simulink model "Experiment1_model"  (R2022a)
settings: Solver=FixedStepAuto  StartTime=0.0  StopTime=20  RelTol=1e-3
libraries: slpidlib x32, slctrlblks x18
(part 5 of 5)

== matlab function Experiment1_model/Safety CBF Enforcement Decentralized with Neighbours /CBF Robot5/Neighbourhood Radius ==
  data: hx5 input; hx5 output; qx5 input; deltaP5 input; qx5 output
function [hx5, qx5] = fcn(hx5, qx5, deltaP5)

E = 7;         % Maximum number of barriers
Ds = 0.6;      % Safe Distance
gamma = 0.3;   % Neighbour radius parameter 

Dn5 = Ds + 1/(2*(10+10)) * ((2*(10+10)/gamma)^(1/2) + (2+2))^2;

for i=1:E
    if deltaP5(i) >= Dn5
        hx5(i) = 0;
        qx5(i,:) = 0;
    end
end

== matlab function Experiment1_model/Safety CBF Enforcement Decentralized with Neighbours /CBF Robot6/DeltaP ==
  data: states input; deltaP6 output
function deltaP6 = fcn(states)

p1 = states(1:2);
p2 = states(3:4);
p3 = states(5:6);
p4 = states(7:8);
p5 = states(9:10);
p6 = states(11:12);
p7 = states(13:14);
p8 = states(15:16);

v1 = states(17:18);
v2 = states(19:20);
v3 = states(21:22);
v4 = states(23:24);
v5 = states(25:26);
v6 = states(27:28);
v7 = states(29:30);
v8 = states(31:32);

deltaP6 = CBF8Robots_deltaP6(states);

== matlab function Experiment1_model/Safety CBF Enforcement Decentralized with Neighbours /CBF Robot6/Neighbourhood Radius ==
  data: hx6 input; hx6 output; qx6 input; deltaP6 input; qx6 output
function [hx6, qx6] = fcn(hx6, qx6, deltaP6)

E = 7;         % Maximum number of barriers
Ds = 0.6;      % Safe Distance
gamma = 0.3;   % Neighbour radius parameter 

Dn6 = Ds + 1/(2*(10+10)) * ((2*(10+10)/gamma)^(1/2) + (2+2))^2;

for i=1:E
    if deltaP6(i) >= Dn6
        hx6(i) = 0;
        qx6(i,:) = 0;
    end
end

== matlab function Experiment1_model/Safety CBF Enforcement Decentralized with Neighbours /CBF Robot7/DeltaP ==
  data: states input; deltaP7 output
function deltaP7 = fcn(states)

p1 = states(1:2);
p2 = states(3:4);
p3 = states(5:6);
p4 = states(7:8);
p5 = states(9:10);
p6 = states(11:12);
p7 = states(13:14);
p8 = states(15:16);

v1 = states(17:18);
v2 = states(19:20);
v3 = states(21:22);
v4 = states(23:24);
v5 = states(25:26);
v6 = states(27:28);
v7 = states(29:30);
v8 = states(31:32);

deltaP7 = CBF8Robots_deltaP7(states);

== matlab function Experiment1_model/Safety CBF Enforcement Decentralized with Neighbours /CBF Robot7/Neighbourhood Radius ==
  data: hx7 input; hx7 output; qx7 input; deltaP7 input; qx7 output
function [hx7, qx7] = fcn(hx7, qx7, deltaP7)

E = 7;         % Maximum number of barriers
Ds = 0.6;      % Safe Distance
gamma = 0.3;   % Neighbour radius parameter 

Dn7 = Ds + 1/(2*(10+10)) * ((2*(10+10)/gamma)^(1/2) + (2+2))^2;

for i=1:E
    if deltaP7(i) >= Dn7
        hx7(i) = 0;
        qx7(i,:) = 0;
    end
end

== matlab function Experiment1_model/Safety CBF Enforcement Decentralized with Neighbours /CBF Robot8/DeltaP ==
  data: states input; deltaP8 output
function deltaP8 = fcn(states)

p1 = states(1:2);
p2 = states(3:4);
p3 = states(5:6);
p4 = states(7:8);
p5 = states(9:10);
p6 = states(11:12);
p7 = states(13:14);
p8 = states(15:16);

v1 = states(17:18);
v2 = states(19:20);
v3 = states(21:22);
v4 = states(23:24);
v5 = states(25:26);
v6 = states(27:28);
v7 = states(29:30);
v8 = states(31:32);

deltaP8 = CBF8Robots_deltaP8(states);

== matlab function Experiment1_model/Safety CBF Enforcement Decentralized with Neighbours /CBF Robot8/Neighbourhood Radius ==
  data: hx8 input; hx8 output; qx8 input; deltaP8 input; qx8 output
function [hx8, qx8] = fcn(hx8, qx8, deltaP8)

E = 7;         % Maximum number of barriers
Ds = 0.6;      % Safe Distance
gamma = 0.3;   % Neighbour radius parameter 

Dn8 = Ds + 1/(2*(10+10)) * ((2*(10+10)/gamma)^(1/2) + (2+2))^2;

for i=1:E
    if deltaP8(i) >= Dn8
        hx8(i) = 0;
        qx8(i,:) = 0;
    end
end

== matlab function Experiment1_model/Safety CBF Enforcement Decentralized with Neighbours /CBF Robot8/dh ==
  data: states input size=32; qx8 output size=[7 4]
function qx8 = fcn(states)
p1 = states(1:2);
p2 = states(3:4);
p3 = states(5:6);
p4 = states(7:8);
p5 = states(9:10);
p6 = states(11:12);
p7 = states(13:14);
p8 = states(15:16);

v1 = states(17:18);
v2 = states(19:20);
v3 = states(21:22);
v4 = states(23:24);
v5 = states(25:26);
v6 = states(27:28);
v7 = states(29:30);
v8 = states(31:32);

qx8 = CBF8Robots_dh8(states);

== matlab function Experiment1_model/Safety CBF Enforcement Decentralized with Neighbours /CBF Robot8/h ==
  data: states input size=32; hx8 output size=7
function hx8 = fcn(states)

p1 = states(1:2);
p2 = states(3:4);
p3 = states(5:6);
p4 = states(7:8);
p5 = states(9:10);
p6 = states(11:12);
p7 = states(13:14);
p8 = states(15:16);

v1 = states(17:18);
v2 = states(19:20);
v3 = states(21:22);
v4 = states(23:24);
v5 = states(25:26);
v6 = states(27:28);
v7 = states(29:30);
v8 = states(31:32);

hx8 = CBF8Robots_h8(states);

== matlab function Experiment1_model/Controller3 PID/Signal Routing ==
  data: states input; x_rob1 output; x_rob2 output; x_rob3 output; x_rob4 output; x_rob5 output; x_rob6 output; x_rob7 output; x_rob8 output
function [x_rob1, x_rob2, x_rob3, x_rob4, x_rob5, x_rob6, x_rob7, x_rob8] = fcn(states)


x_rob1 = [states(1); states(2); states(17); states(18)];
x_rob2 = [states(3); states(4); states(19); states(20)];
x_rob3 = [states(5); states(6); states(21); states(22)];
x_rob4 = [states(7); states(8); states(23); states(24)];
x_rob5 = [states(9); states(10); states(25); states(26)];
x_rob6 = [states(11); states(12); states(27); states(28)];
x_rob7 = [states(13); states(14); states(29); states(30)];
x_rob8 = [states(15); states(16); states(31); states(32)];

== matlab function Experiment1_model/Robots Dynamics Decentralized/Signal Reshaping ==
  data: p1 input; p output; v1 input; p2 input; v2 input; p3 input; v3 input; p4 input; v4 input; p5 input; v5 input; p6 input; v6 input; p7 input; v7 input; p8 input; v8 input; v output
function [p,v] = fcn(p1,v1,p2,v2,p3,v3,p4,v4,p5,v5,p6,v6,p7,v7,p8,v8)

p = [p1;p2;p3;p4;p5;p6;p7;p8;];
v = [v1;v2;v3;v4;v5;v6;v7;v8;];

== matlab function Experiment1_model/Robots Dynamics Decentralized/Visualization/MATLAB Function ==
  data: p input
function fcn(p)
Nrobots = 8;                    % number of robots in simulation
RobotRadius = 0.25;                % desired robot radius
colors = {"red", "blue", "green", "cyan", "magenta", "black", "yellow", "#EDB120"}; %colors

x = [p(1); p(3); p(5); p(7); p(9); p(11); p(13); p(15)];
y = [p(2); p(4); p(6); p(8); p(10); p(12); p(14); p(16)];

StartPos = [x y];




for i=1:Nrobots
    
    % create the ith robot 
    pos = [StartPos(i,:)-RobotRadius 2*RobotRadius 2*RobotRadius]; %position of the robot by considering its radius
    r = rectangle('Position', pos, 'Curvature',[1 1], 'FaceColor', colors{i}, 'Edgecolor','none'); %graph of the robot as it were a kind of circle, for simplicity
    
    axis([-20 20 -20 20]) %axis of the graph: x axis from 0 to 100, the same for y
    title('Robots simulation');
    figure(1); hold on;
    %pause(0.5); 
    
    
    

end

% clf

== matlab function Experiment1_model/Robot Dynamics Centralized /Visualization1/MATLAB Function ==
  data: p input
function fcn(p)
Nrobots = 8;                    % number of robots in simulation
RobotRadius = 0.07;                % desired robot radius
colors = {"blue", "blue", "blue","blue", "blue", "blue", "blue", "blue"}; %colors

x = [p(1); p(3); p(5); p(7); p(9); p(11); p(13); p(15)];
y = [p(2); p(4); p(6); p(8); p(10); p(12); p(14); p(16)];

StartPos = [x y];




for i=1:Nrobots
    
    % create the ith robot 
    pos = [StartPos(i,:)-RobotRadius 2*RobotRadius 2*RobotRadius]; %position of the robot by considering its radius
    r = rectangle('Position', pos, 'Curvature',[1 1], 'FaceColor', colors{i}, 'Edgecolor','none'); %graph of the robot as it were a kind of circle, for simplicity
    
    axis([-11 13 -11 11]) %axis of the graph: x axis from 0 to 100, the same for y
    title('Robots simulation');
    figure(1); hold on;
    %pause(0.5); 
    
    
    

end

% clf

== matlab function Experiment1_model/Robot Dynamics Centralized with Neighbours/Signal Reshaping ==
  data: p1 input; p output; v1 input; p2 input; v2 input; p3 input; v3 input; p4 input; v4 input; p5 input; v5 input; p6 input; v6 input; p7 input; v7 input; p8 input; v8 input; v output
function [p,v] = fcn(p1,v1,p2,v2,p3,v3,p4,v4,p5,v5,p6,v6,p7,v7,p8,v8)

p = [p1;p2;p3;p4;p5;p6;p7;p8;];
v = [v1;v2;v3;v4;v5;v6;v7;v8;];

== matlab function Experiment1_model/Robot Dynamics Centralized with Neighbours/Visualization/MATLAB Function ==
  data: p input
function fcn(p)
Nrobots = 8;                    % number of robots in simulation
RobotRadius = 0.25;                % desired robot radius
colors = {"red", "blue", "green", "cyan", "magenta", "black", "yellow", "#EDB120"}; %colors

x = [p(1); p(3); p(5); p(7); p(9); p(11); p(13); p(15)];
y = [p(2); p(4); p(6); p(8); p(10); p(12); p(14); p(16)];

StartPos = [x y];




for i=1:Nrobots
    
    % create the ith robot 
    pos = [StartPos(i,:)-RobotRadius 2*RobotRadius 2*RobotRadius]; %position of the robot by considering its radius
    r = rectangle('Position', pos, 'Curvature',[1 1], 'FaceColor', colors{i}, 'Edgecolor','none'); %graph of the robot as it were a kind of circle, for simplicity
    
    axis([-20 20 -20 20]) %axis of the graph: x axis from 0 to 100, the same for y
    title('Robots simulation');
    figure(1); hold on;
    %pause(0.5); 
    
    
    

end

% clf

== matlab function Experiment1_model/Controller2 PID/Signal Routing ==
  data: states input; x_rob1 output; x_rob2 output; x_rob3 output; x_rob4 output; x_rob5 output; x_rob6 output; x_rob7 output; x_rob8 output
function [x_rob1, x_rob2, x_rob3, x_rob4, x_rob5, x_rob6, x_rob7, x_rob8] = fcn(states)


x_rob1 = [states(1); states(2); states(17); states(18)];
x_rob2 = [states(3); states(4); states(19); states(20)];
x_rob3 = [states(5); states(6); states(21); states(22)];
x_rob4 = [states(7); states(8); states(23); states(24)];
x_rob5 = [states(9); states(10); states(25); states(26)];
x_rob6 = [states(11); states(12); states(27); states(28)];
x_rob7 = [states(13); states(14); states(29); states(30)];
x_rob8 = [states(15); states(16); states(31); states(32)];

== matlab function Experiment1_model/Robots Dynamics Decentralized1/Signal Reshaping ==
  data: p1 input; p output; v1 input; p2 input; v2 input; p3 input; v3 input; p4 input; v4 input; p5 input; v5 input; p6 input; v6 input; p7 input; v7 input; p8 input; v8 input; v output
function [p,v] = fcn(p1,v1,p2,v2,p3,v3,p4,v4,p5,v5,p6,v6,p7,v7,p8,v8)

p = [p1;p2;p3;p4;p5;p6;p7;p8;];
v = [v1;v2;v3;v4;v5;v6;v7;v8;];

== matlab function Experiment1_model/Robots Dynamics Decentralized1/Visualization/MATLAB Function ==
  data: p input
function fcn(p)
Nrobots = 8;                    % number of robots in simulation
RobotRadius = 0.25;                % desired robot radius
colors = {"red", "blue", "green", "cyan", "magenta", "black", "yellow", "#EDB120"}; %colors

x = [p(1); p(3); p(5); p(7); p(9); p(11); p(13); p(15)];
y = [p(2); p(4); p(6); p(8); p(10); p(12); p(14); p(16)];

StartPos = [x y];




for i=1:Nrobots
    
    % create the ith robot 
    pos = [StartPos(i,:)-RobotRadius 2*RobotRadius 2*RobotRadius]; %position of the robot by considering its radius
    r = rectangle('Position', pos, 'Curvature',[1 1], 'FaceColor', colors{i}, 'Edgecolor','none'); %graph of the robot as it were a kind of circle, for simplicity
    
    axis([-20 20 -20 20]) %axis of the graph: x axis from 0 to 100, the same for y
    title('Robots simulation');
    figure(1); hold on;
    %pause(0.5); 
    
    
    

end

% clf

== matlab function Experiment1_model/Robot Dynamics Centralized /Visualization/MATLAB Function ==
  data: p input
function fcn(p)
Nrobots = 8;                    % number of robots in simulation
RobotRadius = 0.25;                % desired robot radius
colors = {"red", "blue", "green", "cyan", "magenta", "black", "yellow", "#EDB120"}; %colors

x = [p(1); p(3); p(5); p(7); p(9); p(11); p(13); p(15)];
y = [p(2); p(4); p(6); p(8); p(10); p(12); p(14); p(16)];

StartPos = [x y];




for i=1:Nrobots
    
    % create the ith robot 
    pos = [StartPos(i,:)-RobotRadius 2*RobotRadius 2*RobotRadius]; %position of the robot by considering its radius
    r = rectangle('Position', pos, 'Curvature',[1 1], 'FaceColor', colors{i}, 'Edgecolor','none'); %graph of the robot as it were a kind of circle, for simplicity
    
    axis([-20 20 -20 20]) %axis of the graph: x axis from 0 to 100, the same for y
    title('Robots simulation');
    figure(1); hold on;
    %pause(0.5); 
    
    
    

end

% clf

== matlab function Experiment1_model/Controller3 PID1/Signal Routing ==
  data: states input; x_rob1 output; x_rob2 output; x_rob3 output; x_rob4 output; x_rob5 output; x_rob6 output; x_rob7 output; x_rob8 output
function [x_rob1, x_rob2, x_rob3, x_rob4, x_rob5, x_rob6, x_rob7, x_rob8] = fcn(states)


x_rob1 = [states(1); states(2); states(17); states(18)];
x_rob2 = [states(3); states(4); states(19); states(20)];
x_rob3 = [states(5); states(6); states(21); states(22)];
x_rob4 = [states(7); states(8); states(23); states(24)];
x_rob5 = [states(9); states(10); states(25); states(26)];
x_rob6 = [states(11); states(12); states(27); states(28)];
x_rob7 = [states(13); states(14); states(29); states(30)];
x_rob8 = [states(15); states(16); states(31); states(32)];

== matlab function Experiment1_model/Robot Dynamics Centralized with Neighbours/Visualization1/MATLAB Function ==
  data: p input
function fcn(p)
Nrobots = 8;                    % number of robots in simulation
RobotRadius = 0.07;                % desired robot radius
colors = {"green","green", "green", "green", "green", "green", "green", "green"}; %colors

x = [p(1); p(3); p(5); p(7); p(9); p(11); p(13); p(15)];
y = [p(2); p(4); p(6); p(8); p(10); p(12); p(14); p(16)];

StartPos = [x y];




for i=1:Nrobots
    
    % create the ith robot 
    pos = [StartPos(i,:)-RobotRadius 2*RobotRadius 2*RobotRadius]; %position of the robot by considering its radius
    r = rectangle('Position', pos, 'Curvature',[1 1], 'FaceColor', colors{i}, 'Edgecolor','none'); %graph of the robot as it were a kind of circle, for simplicity
    
    axis([-11 13 -11 11]) %axis of the graph: x axis from 0 to 100, the same for y
    title('Robots simulation');
    figure(1); hold on;
    %pause(0.5); 
    
    
    

end

% clf

== matlab function Experiment1_model/Robots Dynamics Decentralized/Visualization1/MATLAB Function ==
  data: p input
function fcn(p)
Nrobots = 8;                    % number of robots in simulation
RobotRadius = 0.07;                % desired robot radius
colors = {"red","red", "red", "red", "red", "red", "red", "red"}; %colors

x = [p(1); p(3); p(5); p(7); p(9); p(11); p(13); p(15)];
y = [p(2); p(4); p(6); p(8); p(10); p(12); p(14); p(16)];

StartPos = [x y];




for i=1:Nrobots
    
    % create the ith robot 
    pos = [StartPos(i,:)-RobotRadius 2*RobotRadius 2*RobotRadius]; %position of the robot by considering its radius
    r = rectangle('Position', pos, 'Curvature',[1 1], 'FaceColor', colors{i}, 'Edgecolor','none'); %graph of the robot as it were a kind of circle, for simplicity
    
    axis([-11 13 -11 11]) %axis of the graph: x axis from 0 to 100, the same for y
    title('Robots simulation');
    figure(1); hold on;
    %pause(0.5); 
    
    
    

end

% clf

== matlab function Experiment1_model/Robots Dynamics Decentralized1/Visualization1/MATLAB Function ==
  data: p input
function fcn(p)
Nrobots = 8;                    % number of robots in simulation
RobotRadius = 0.07;                % desired robot radius
colors = {"yellow", "yellow", "yellow", "yellow", "yellow", "yellow", "yellow", "yellow"}; %colors

x = [p(1); p(3); p(5); p(7); p(9); p(11); p(13); p(15)];
y = [p(2); p(4); p(6); p(8); p(10); p(12); p(14); p(16)];

StartPos = [x y];




for i=1:Nrobots
    
    % create the ith robot 
    pos = [StartPos(i,:)-RobotRadius 2*RobotRadius 2*RobotRadius]; %position of the robot by considering its radius
    r = rectangle('Position', pos, 'Curvature',[1 1], 'FaceColor', colors{i}, 'Edgecolor','none'); %graph of the robot as it were a kind of circle, for simplicity
    
    axis([-11 13 -11 11]) %axis of the graph: x axis from 0 to 100, the same for y
    title('Robots simulation');
    figure(1); hold on;
    %pause(0.5); 
    
    
    

end

% clf

== matlab function Experiment1_model/Safety CBF Enforcement Centralized /h ==
  data: states input size=32; hx output size=28
function hx = fcn(states)

p1 = states(1:2);
p2 = states(3:4);
p3 = states(5:6);
p4 = states(7:8);
p5 = states(9:10);
p6 = states(11:12);
p7 = states(13:14);
p8 = states(15:16);

v1 = states(17:18);
v2 = states(19:20);
v3 = states(21:22);
v4 = states(23:24);
v5 = states(25:26);
v6 = states(27:28);
v7 = states(29:30);
v8 = states(31:32);

hx = CBF8Robots_h(states);

== matlab function Experiment1_model/Safety CBF Enforcement Centralized /dh ==
  data: states input size=32; qx output size=[28 32]
function qx = fcn(states)
p1 = states(1:2);
p2 = states(3:4);
p3 = states(5:6);
p4 = states(7:8);
p5 = states(9:10);
p6 = states(11:12);
p7 = states(13:14);
p8 = states(15:16);

v1 = states(17:18);
v2 = states(19:20);
v3 = states(21:22);
v4 = states(23:24);
v5 = states(25:26);
v6 = states(27:28);
v7 = states(29:30);
v8 = states(31:32);

qx = CBF8Robots_dh(states);

== matlab function Experiment1_model/Safety CBF Enforcement Centralized with Neighbours /DeltaP ==
  data: states input; deltaP output
function deltaP = fcn(states)

p1 = states(1:2);
p2 = states(3:4);
p3 = states(5:6);
p4 = states(7:8);
p5 = states(9:10);
p6 = states(11:12);
p7 = states(13:14);
p8 = states(15:16);

v1 = states(17:18);
v2 = states(19:20);
v3 = states(21:22);
v4 = states(23:24);
v5 = states(25:26);
v6 = states(27:28);
v7 = states(29:30);
v8 = states(31:32);

deltaP = CBF8Robots_deltaP(states);

== matlab function Experiment1_model/Safety CBF Enforcement Decentralized /CBF Robot1/dh ==
  data: states input size=32; qx1 output size=[7 4]
function qx1 = fcn(states)
p1 = states(1:2);
p2 = states(3:4);
p3 = states(5:6);
p4 = states(7:8);
p5 = states(9:10);
p6 = states(11:12);
p7 = states(13:14);
p8 = states(15:16);

v1 = states(17:18);
v2 = states(19:20);
v3 = states(21:22);
v4 = states(23:24);
v5 = states(25:26);
v6 = states(27:28);
v7 = states(29:30);
v8 = states(31:32);

qx1 = CBF8Robots_dh1(states);

== matlab function Experiment1_model/Safety CBF Enforcement Decentralized /CBF Robot1/h ==
  data: states input size=32; hx1 output size=7
function hx1 = fcn(states)

p1 = states(1:2);
p2 = states(3:4);
p3 = states(5:6);
p4 = states(7:8);
p5 = states(9:10);
p6 = states(11:12);
p7 = states(13:14);
p8 = states(15:16);

v1 = states(17:18);
v2 = states(19:20);
v3 = states(21:22);
v4 = states(23:24);
v5 = states(25:26);
v6 = states(27:28);
v7 = states(29:30);
v8 = states(31:32);

hx1 = CBF8Robots_h1(states);
